simulink model "FlwPthChar_TestBed_org"  (Simulink 10.0)
settings: Solver=FixedStepDiscrete  StartTime=0.0  StopTime=1  FixedStep=1  RelTol=1e-3  EnableMultiTasking=on
undefined symbols (not defined in the file): MWS
libraries: Lib_Turbo_FlowPathChar_TMATS x1
settings Model: Creator=jwchapm2  LastModifiedBy=annonymous
settings DataIOCC: LimitDataPoints=on
settings OptimizationCC: ExpressionDepthLimit=2147483647
settings DebuggingCC: SolverPrmCheckMsg=warning  StateNameClashWarn=warning
settings GRTTargetCC: GeneratePreprocessorConditionals=Disable all  CombineOutputUpdateFcns=on  GRTInterface=off
settings ConfigComp: CovExternalEMLEnable=off

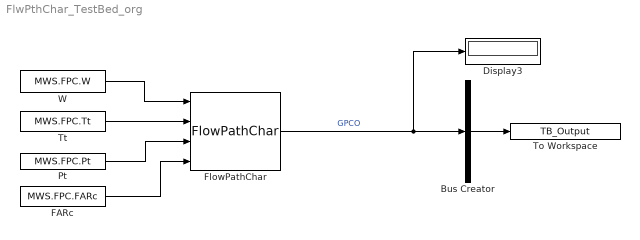
== system FlwPthChar_TestBed_org ==
  Bus Creator : BusCreator  Inputs=1
  Display3 : Display
  FARc : Constant  Value=MWS.FPC.FARc
  FlowPathChar : Lib_Turbo_FlowPathChar_TMATS/FlowPathChar
  Pt : Constant  Value=MWS.FPC.Pt
  To Workspace : ToWorkspace  VariableName=TB_Output  SampleTime=-1
  Tt : Constant  Value=MWS.FPC.Tt
  W : Constant  Value=MWS.FPC.W
  wires:
  W/1 -> FlowPathChar/1
  FARc/1 -> FlowPathChar/4
  Tt/1 -> FlowPathChar/2
  Pt/1 -> FlowPathChar/3
  FlowPathChar/1 -> Display3/1, Bus Creator/1  "GPCO"
  Bus Creator/1 -> To Workspace/1
